simulink model "etc_benchTest"  (R2019b)
settings: Solver=FixedStepDiscrete  StartTime=0.0  StopTime=Inf  RelTol=1e-3  EnableMultiTasking=on
PreLoadFcn:
  | RTWConfigurationCB('preloadfcn', bdroot);
undefined symbols (not defined in the file or in its folder): __PRM__SERIALIZED__DATA__, SubsystemReferenceBlock
libraries: simulink x2, c280xlib x1
settings Model: DataDictionary=etc_benchTest.sldd  ExtModeTrigDuration=8  OrderedModelArguments=off  Creator=Nick  LastModifiedBy=Nick
settings OptimizationCC: DefaultUnderspecifiedDataType=single  EnhancedBackFolding=on  PassReuseOutputArgsAs=Individual arguments  ZeroExternalMemoryAtStartup=off  MaxStackSize=1024  OptimizeBlockOrder=speed  DifferentSizesBufferReuse=on  OptimizationCustomize=off  DenormalBehavior=FlushToZero  EfficientTunableParamExpr=on
settings DebuggingCC: ParameterTunabilityLossMsg=error  UnitsInconsistencyMsg=none
settings HardwareCC: ProdBitPerChar=16  ProdBitPerInt=16  ProdBitPerPointer=32  ProdBitPerSizeT=32  ProdBitPerPtrDiffT=32  ProdLargestAtomicInteger=Integer  ProdLargestAtomicFloat=None  ProdWordSize=16  ProdHWDeviceType=Texas Instruments->C2000
settings SFSimCC: MATLABDynamicMemAlloc=off
settings RTWCC: SystemTargetFile=ert.tlc  HardwareBoard=TI Delfino F28377S LaunchPad  TLCOptions=-aInlineSetEventsForThisBaseRateFcn=TLC_FALSE -aSuppressMultiTaskScheduler=TLC_FALSE -aRateBasedStepFcn=1  TemplateMakefile=ert_default_tmf  GenerateReport=on  Toolchain=Texas Instruments Code Composer Studio (C2000)  IncludeHyperlinkInReport=on  LaunchReport=on  GenerateTraceInfo=on  GenerateTraceReport=on  GenerateTraceReportSl=on  GenerateTraceReportSf=on  GenerateTraceReportEml=on
settings CodeAppCC: ForceParamTrailComments=on  IgnoreCustomStorageClasses=off  OperatorAnnotations=on  SimulinkDataObjDesc=on  SFDataObjDesc=on  InsertBlockDesc=on
settings ERTTargetCC: TargetLangStandard=C99 (ISO)  CodeReplacementLibrary=TI C28x  GenerateASAP2=on  ExtModeStaticAllocSize=10000  RootIOFormat=Structure reference

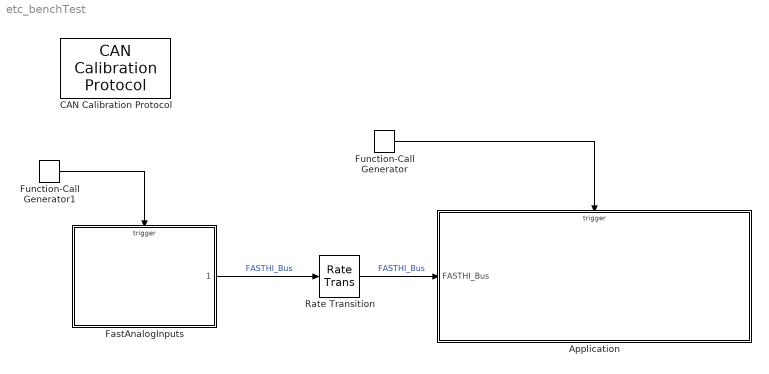
== system etc_benchTest ==
  Application : Subsystem
  CAN Calibration Protocol : c280xlib/CAN Calibration Protocol  CCP_STATION_ID=hex2dec('1')  module=eCAN_A  ccp_cro_id=hex2dec('6FA')  ccp_cro_message_type=Extended (29-bit identifier)  ccp_return_id=hex2dec('6FB')  ccp_return_message_type=Extended (29-bit identifier)  TOTAL_NUM_ODTS=20  cro_sample_time=0.1
      settings: SourceProductName=Embedded Coder Support Package for Texas Instruments C2000 Processors  SourceProductBaseCode=TIC2000
  FastAnalogInputs : Subsystem  BlockKeywords=__PRM__SERIALIZED__DATA__:SubsystemReferenceBlock  ReferencedSubsystem=HI_FastAnalogInputs
  Function-Call Generator : simulink/Ports & Subsystems/Function-Call Generator  sample_time=.001  numberOfIterations=1
  Function-Call Generator1 : simulink/Ports & Subsystems/Function-Call Generator  sample_time=.00001  numberOfIterations=1
  Rate Transition : RateTransition
  wires:
  Function-Call Generator/1 -> Application/Trigger
  FastAnalogInputs/1 -> Rate Transition/1  "FASTHI_Bus"
  Function-Call Generator1/1 -> FastAnalogInputs/Trigger
  Rate Transition/1 -> Application/1(FASTHI_Bus)  "FASTHI_Bus"

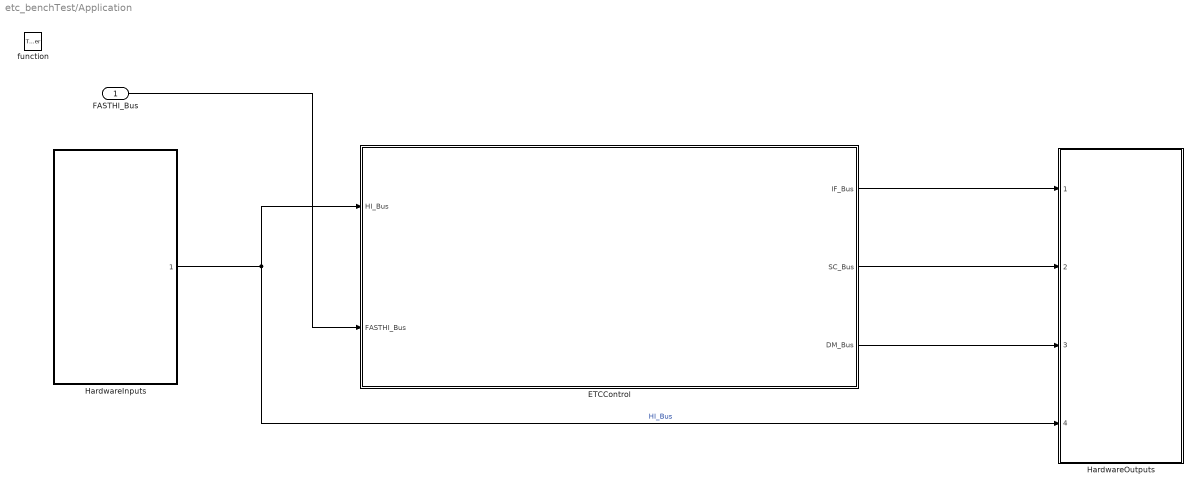
== system etc_benchTest/Application ==
  FASTHI_Bus : Inport
  function : TriggerPort  TriggerType=function-call  VariantControl=Variant
  ETCControl : Subsystem
  HardwareInputs : Subsystem  BlockKeywords=__PRM__SERIALIZED__DATA__:SubsystemReferenceBlock  ReferencedSubsystem=HardwareInputs
  HardwareOutputs : Subsystem  BlockKeywords=__PRM__SERIALIZED__DATA__:SubsystemReferenceBlock  ReferencedSubsystem=HardwareOutputs
  wires:
  HardwareInputs/1 -> HardwareOutputs/4, ETCControl/1(HI_Bus)  "HI_Bus"
  ETCControl/1(IF_Bus) -> HardwareOutputs/1
  ETCControl/2(SC_Bus) -> HardwareOutputs/2
  ETCControl/3(DM_Bus) -> HardwareOutputs/3
  FASTHI_Bus/1 -> ETCControl/2(FASTHI_Bus)

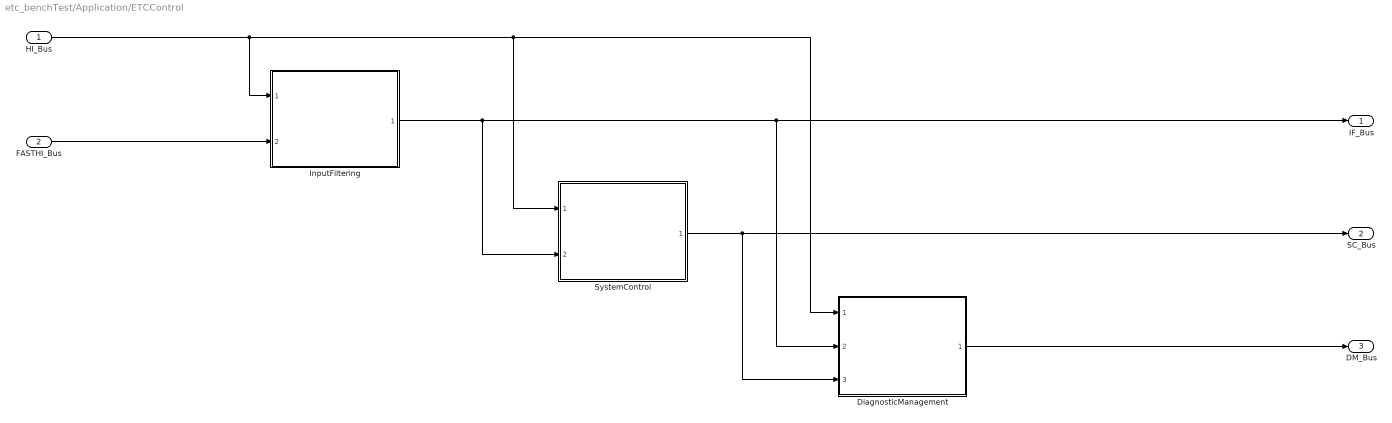
== system etc_benchTest/Application/ETCControl ==
  HI_Bus : Inport
  FASTHI_Bus : Inport  Port=2
  DiagnosticManagement : Subsystem  BlockKeywords=__PRM__SERIALIZED__DATA__:SubsystemReferenceBlock  ReferencedSubsystem=DiagnosticManagement
  InputFiltering : Subsystem  BlockKeywords=__PRM__SERIALIZED__DATA__:SubsystemReferenceBlock  ReferencedSubsystem=InputFiltering
  SystemControl : Subsystem  BlockKeywords=__PRM__SERIALIZED__DATA__:SubsystemReferenceBlock  ReferencedSubsystem=SystemControl
  IF_Bus : Outport
  SC_Bus : Outport  Port=2
  DM_Bus : Outport  Port=3
  wires:
  HI_Bus/1 -> InputFiltering/1, SystemControl/1, DiagnosticManagement/1
  InputFiltering/1 -> IF_Bus/1, DiagnosticManagement/2, SystemControl/2
  SystemControl/1 -> SC_Bus/1, DiagnosticManagement/3
  DiagnosticManagement/1 -> DM_Bus/1
  FASTHI_Bus/1 -> InputFiltering/2
